simulink model "simulink_basic_lab"  (R2022a)
settings: Solver=VariableStepAuto  StartTime=0.0  StopTime=5  RelTol=1e-3
settings Model: Creator=Laptop-Academy.com  LastModifiedBy=Laptop-Academy.com
settings OptimizationCC: DefaultParameterBehavior=Inlined  EnhancedBackFolding=on  PassReuseOutputArgsAs=Individual arguments  ZeroExternalMemoryAtStartup=off  ZeroInternalMemoryAtStartup=off  OptimizeBlockOrder=speed  DifferentSizesBufferReuse=on  OptimizationCustomize=off  EfficientTunableParamExpr=on
settings DebuggingCC: ParameterTunabilityLossMsg=error
settings SFSimCC: MATLABDynamicMemAlloc=off
settings RTWCC: SystemTargetFile=ert.tlc  TemplateMakefile=ert_default_tmf
settings CodeAppCC: ForceParamTrailComments=on  IgnoreCustomStorageClasses=off  OperatorAnnotations=on  SimulinkDataObjDesc=on  SFDataObjDesc=on  InsertBlockDesc=on
settings ERTTargetCC: TargetLangStandard=C99 (ISO)  GenerateSampleERTMain=on  InlinedParameterPlacement=NonHierarchical  ERTCustomFileTemplate=example_file_process.tlc

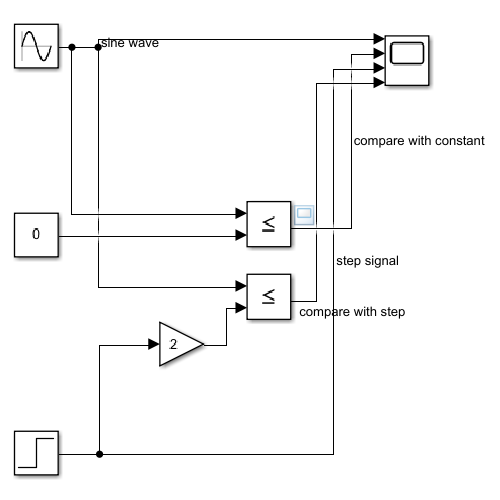
[thumbnail: Simulink's stored preview of the top-level diagram]
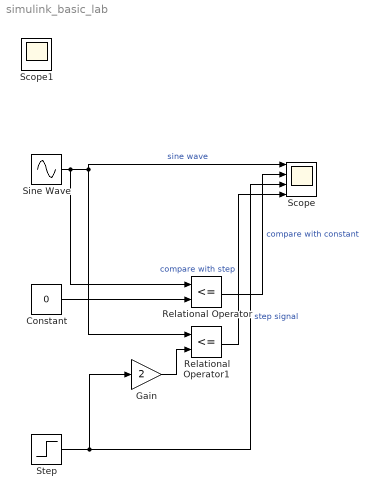
== system simulink_basic_lab ==
  Constant : Constant  Value=0
  Gain : Gain  Gain=2
  Relational Operator : RelationalOperator  Operator=<=  OutDataTypeStr=boolean  RndMeth=Simplest  InputSameDT=off
  Relational Operator1 : RelationalOperator  Operator=<=  OutDataTypeStr=boolean  RndMeth=Simplest  InputSameDT=off
  Scope : Scope  NumInputPorts=4
  Sine Wave : Sin  Frequency=6.2831853  SampleTime=0
  Step : Step  Time=2  SampleTime=2
  Scope1 : Scope
  wires:
  Sine Wave/1 -> Relational Operator/1, Relational Operator1/1, Scope/1  "sine wave"
  Constant/1 -> Relational Operator/2
  Relational Operator/1 -> Scope/2  "compare with constant"
  Step/1 -> Gain/1, Scope/3  "step signal"
  Gain/1 -> Relational Operator1/2
  Relational Operator1/1 -> Scope/4  "compare with step"
